simulink model "simul1_error_space"  (R2022b)
settings: Solver=FixedStepAuto  StartTime=0.0  StopTime=20  FixedStep=0.001  RelTol=1e-3
undefined symbols (not defined in the file): degs2rpm, der, National_Instruments, PCI, rpm2rads, sens, simul, ssError, Ts
libraries: sldrtlib x3
settings Model: SimulationMode=external  ExtModeTrigDuration=50001  ExtModeTrigDurationFloating=50001  Creator=perondavid  LastModifiedBy=david
settings DataIOCC: LoggingToFile=on
settings HardwareCC: ProdBitPerLong=64  ProdHWDeviceType=Intel->x86-64 (Linux 64)
settings RTWCC: Description=Simulink Desktop Real-Time  SystemTargetFile=sldrt.tlc  TemplateMakefile=sldrt.tmf  RTWCompilerOptimization=on
settings CodeAppCC: MaxIdLength=95
settings SimulinkDesktopRealTimeCC: TargetLibSuffix=_sldrt.a  TargetPreCompLibLocation=C:\Program Files\MATLAB\R2022b\toolbox\sldrt\lib\win64

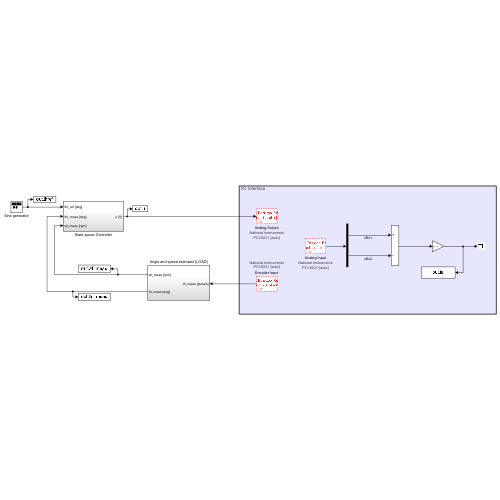
[thumbnail: Simulink's stored preview of the top-level diagram]
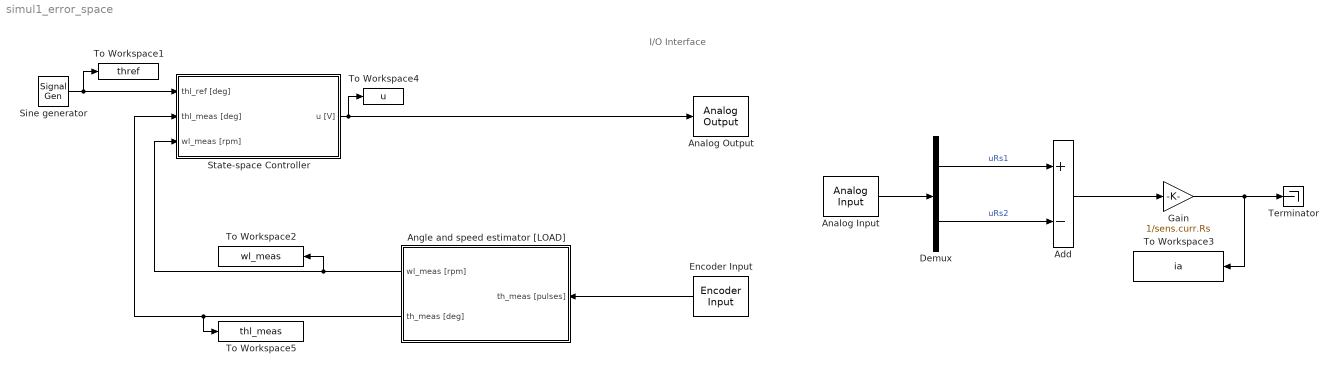
== system simul1_error_space ==
  note: I/O Interface
  Add : Sum  Inputs=+-
  Analog Input : sldrtlib/Analog Input  SampleTime=-1  MaxMissedTicks=10  ShowMissedTicks=off  YieldWhenWaiting=off  DrvName=National_Instruments/PCI-6221  DrvAddress=4294967295  DrvOptions=[0 0 0 2 0]  Channels=[1, 2]  RangeMode=1  VoltRange=1  DataType=1
      settings: AttributesFormatString=National Instruments\nPCI-6221 [auto]
  Analog Output : sldrtlib/Analog Output  SampleTime=-1  MaxMissedTicks=10  ShowMissedTicks=off  YieldWhenWaiting=off  DrvName=National_Instruments/PCI-6221  DrvAddress=4294967295  DrvOptions=[0 0 0 2 0]  Channels=1  RangeMode=1  VoltRange=1  InitialValue=0  FinalValue=0
      settings: AttributesFormatString=National Instruments\nPCI-6221 [auto]
  Angle and speed estimator [LOAD] : Subsystem
  Demux : Demux  Outputs=2
  Encoder Input : sldrtlib/Encoder Input  SampleTime=-1  MaxMissedTicks=10  ShowMissedTicks=off  YieldWhenWaiting=off  DrvName=National_Instruments/PCI-6221  DrvAddress=4294967295  DrvOptions=[0 0 0 2 0]  Channels=1  QuadMode=3  IndexPulse=1  InputFilter=Inf  DataType=1
      settings: AttributesFormatString=National Instruments\nPCI-6221 [auto]
  Gain : Gain  Gain=1/sens.curr.Rs
  Sine generator : SignalGenerator  Amplitude=ssError.amp  Frequency=ssError.freq  Units=rad/sec
  State-space Controller : Subsystem
  Terminator : Terminator
  To Workspace1 : ToWorkspace  VariableName=thref  SaveFormat=Structure With Time  SampleTime=Ts
  To Workspace2 : ToWorkspace  VariableName=wl_meas  SaveFormat=Structure With Time  SampleTime=Ts
  To Workspace3 : ToWorkspace  VariableName=ia  SaveFormat=Structure With Time  SampleTime=Ts
  To Workspace4 : ToWorkspace  VariableName=u  SaveFormat=Structure With Time  SampleTime=Ts
  To Workspace5 : ToWorkspace  VariableName=thl_meas  SaveFormat=Structure With Time  SampleTime=Ts
  wires:
  Demux/1 -> Add/1  "uRs1"
  Demux/2 -> Add/2  "uRs2"
  Add/1 -> Gain/1
  Gain/1 -> To Workspace3/1, Terminator/1
  Analog Input/1 -> Demux/1
  Angle and speed estimator [LOAD]/2(th_meas [deg]) -> To Workspace5/1, State-space Controller/2(thl_meas [deg])
  State-space Controller/1(u [V]) -> Analog Output/1, To Workspace4/1
  Angle and speed estimator [LOAD]/1(wl_meas [rpm]) -> To Workspace2/1, State-space Controller/3(wl_meas [rpm])
  Sine generator/1 -> To Workspace1/1, State-space Controller/1(thl_ref [deg])
  Encoder Input/1 -> Angle and speed estimator [LOAD]/1(th_meas [pulses])

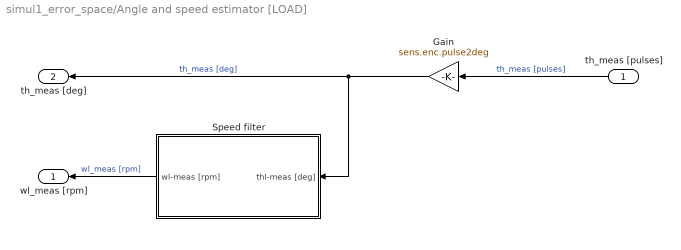
== system simul1_error_space/Angle and speed estimator [LOAD] ==
  th_meas [pulses] : Inport
  Gain : Gain  Gain=sens.enc.pulse2deg
  Speed filter : Subsystem
  wl_meas [rpm] : Outport
  th_meas [deg] : Outport  Port=2
  wires:
  Speed filter/1(wl-meas [rpm]) -> wl_meas [rpm]/1  "wl_meas [rpm]"
  th_meas [pulses]/1 -> Gain/1  "th_meas [pulses]"
  Gain/1 -> Speed filter/1(thl-meas [deg]), th_meas [deg]/1  "th_meas [deg]"

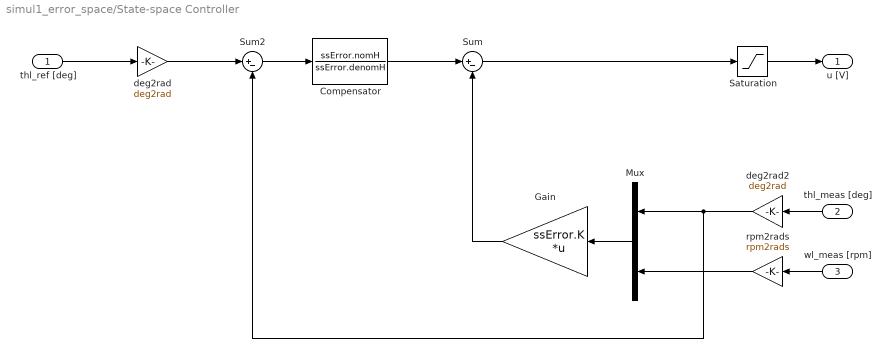
== system simul1_error_space/State-space Controller ==
  thl_ref [deg] : Inport
  thl_meas [deg] : Inport  Port=2
  wl_meas [rpm] : Inport  Port=3
  Compensator : TransferFcn  Numerator=ssError.nomH  Denominator=ssError.denomH
  Gain : Gain  Gain=ssError.K  Multiplication=Matrix(K*u)
  Mux : Mux  Inputs=2
  Saturation : Saturate  UpperLimit=10  LowerLimit=-10
  Sum : Sum  Inputs=|+-
  Sum2 : Sum  Inputs=|+-
  deg2rad : Gain  Gain=deg2rad
  deg2rad2 : Gain  Gain=deg2rad
  rpm2rads : Gain  Gain=rpm2rads
  u [V] : Outport
  wires:
  thl_meas [deg]/1 -> deg2rad2/1
  wl_meas [rpm]/1 -> rpm2rads/1
  Mux/1 -> Gain/1
  thl_ref [deg]/1 -> deg2rad/1
  deg2rad/1 -> Sum2/1
  Sum/1 -> Saturation/1
  deg2rad2/1 -> Mux/1, Sum2/2
  rpm2rads/1 -> Mux/2
  Saturation/1 -> u [V]/1
  Sum2/1 -> Compensator/1
  Compensator/1 -> Sum/1
  Gain/1 -> Sum/2

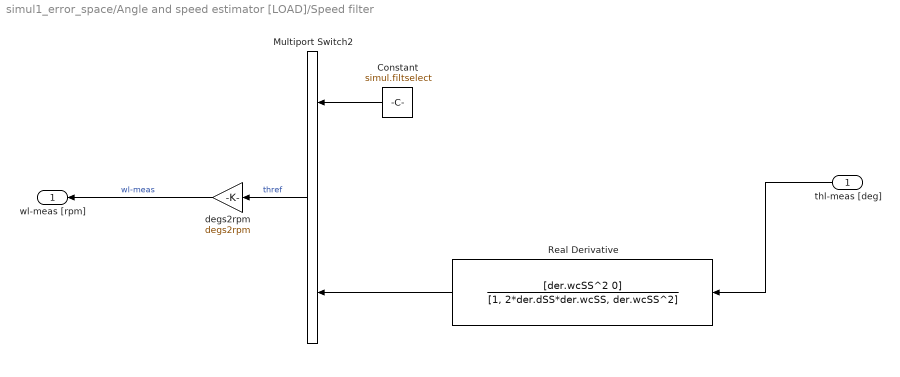
== system simul1_error_space/Angle and speed estimator [LOAD]/Speed filter ==
  thl-meas [deg] : Inport
  Constant : Constant  Value=simul.filtselect
  Multiport Switch2 : MultiPortSwitch  Inputs=2  SaturateOnIntegerOverflow=off  InputSameDT=off
  Real Derivative : TransferFcn  Numerator=[der.wcSS^2 0]  Denominator=[1, 2*der.dSS*der.wcSS, der.wcSS^2]
  degs2rpm : Gain  Gain=degs2rpm
  wl-meas [rpm] : Outport
  wires:
  degs2rpm/1 -> wl-meas [rpm]/1  "wl-meas"
  Real Derivative/1 -> Multiport Switch2/3
  Multiport Switch2/1 -> degs2rpm/1  "thref"
  Constant/1 -> Multiport Switch2/1
  thl-meas [deg]/1 -> Real Derivative/1
